simulink model "PercobaanElinKu"  (R2021a)
settings: Solver=VariableStepAuto  StartTime=0.0  StopTime=10.0  RelTol=1e-3
values from neighbouring files (symbols this model uses):
  F = 500    [JeremyElin.m]    (also in TugasElink.m = 1; UTS.m = 20; tgs.m = 20)
  k = 2000000    [JeremyElin.m]    (also in JeremyElin_K.m = 1; PercobaanElin.m = 1.3862; Riswari.m; TugasElink.m = 1)
undefined symbols (not defined in the file or in its folder): hv
libraries: pid_lib x1
settings Model: Creator=asus  LastModifiedBy=asus

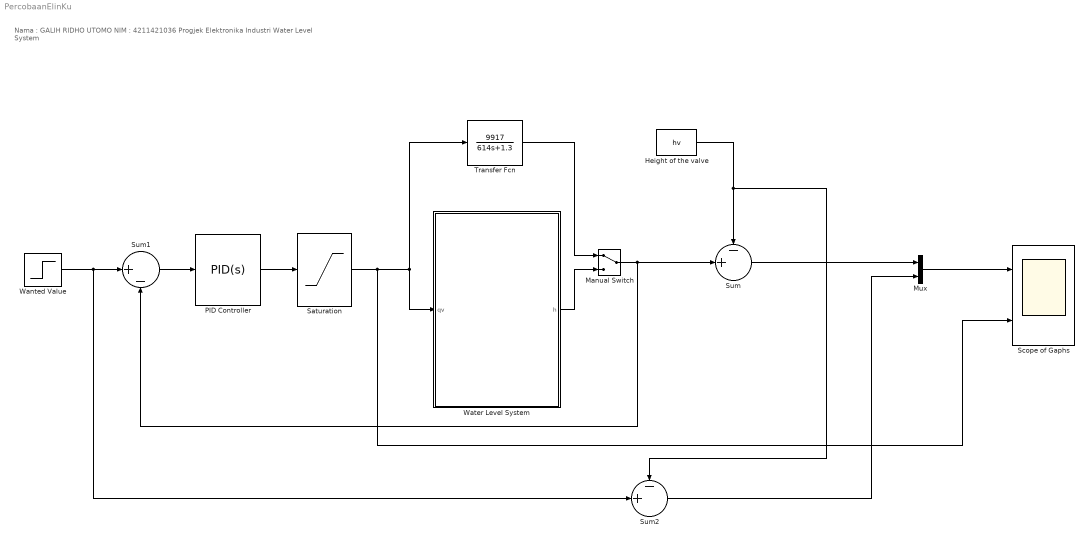
== system PercobaanElinKu ==
  note: Nama 	: GALIH RIDHO UTOMO
      | NIM 	: 4211421036
      | Progjek Elektronika Industri Water Level System
  Height of the valve : Constant  Value=hv
  Manual Switch : ManualSwitch
  Mux : Mux  Inputs=2
  PID Controller : pid_lib/PID Controller  Controller=PID  Form=Parallel  TimeDomain=Continuous-time  UseExternalTs=off  SampleTime=-1  IntegratorMethod=Forward Euler  FilterMethod=Forward Euler  ControllerParametersSource=internal  P=0.000714425130471728  I=3.53685623964158e-06  D=-0.0103917451728758  UseFilter=on  N=0.0336580030389097  TunerSelectOption=Transfer Function Based (PID Tuner App)  InitialConditionSource=internal  InitialConditionForIntegrator=0  InitialConditionForFilter=0  DifferentiatorICPrevScaledInput=0  ExternalReset=none  TrackingMode=off  Kt=1  LimitOutput=off  SatLimitsSource=internal  UpperSaturationLimit=inf  LowerSaturationLimit=-inf  LinearizeAsGain=on  AntiWindupMode=none  Kb=1  POutMin=[]  POutMax=[]  IOutMin=[]  IOutMax=[]  DOutMin=[]  DOutMax=[]  NOutMin=[]  NOutMax=[]  SumOutMin=[]  SumOutMax=[]  SaturationOutMin=[]  SaturationOutMax=[]  PParamMin=[]  PParamMax=[]  IParamMin=[]  IParamMax=[]  DParamMin=[]  DParamMax=[]  NParamMin=[]  NParamMax=[]  KbParamMin=[]  KbParamMax=[]  KtParamMin=[]  KtParamMax=[]  KbOutMin=[]  KbOutMax=[]  KtOutMin=[]  KtOutMax=[]  IntegratorOutMin=[]  IntegratorOutMax=[]  FilterOutMin=[]  FilterOutMax=[]  SumI1OutMin=[]  SumI1OutMax=[]  SumI2OutMin=[]  SumI2OutMax=[]  SumI3OutMin=[]  SumI3OutMax=[]  SumI4OutMin=[]  SumI4OutMax=[]  SumDOutMin=[]  SumDOutMax=[]  DifferentiatorOutMin=[]  DifferentiatorOutMax=[]  FilterDiffOutCoefMin=[]  FilterDiffOutCoefMax=[]  ReciprocalOutMin=[]  ReciprocalOutMax=[]  SumDenOutMin=[]  SumDenOutMax=[]  SumNumOutMin=[]  SumNumOutMax=[]  DivideOutMin=[]  DivideOutMax=[]  UdiffTsProdOutMin=[]  UdiffTsProdOutMax=[]  NTsProdOutMin=[]  NTsProdOutMax=[]  UintegralTsProdOutMin=[]  UintegralTsProdOutMax=[]  UngainTsProdOutMin=[]  UngainTsProdOutMax=[]  IntegratorContinuousStateAttributes=''  IntegratorStateMustResolveToSignalObject=off  IntegratorRTWStateStorageClass=Auto  FilterContinuousStateAttributes=''  FilterStateMustResolveToSignalObject=off  FilterRTWStateStorageClass=Auto  ParallelPVariant=InternalParameters  IdealPVariant=Disabled  IVariant=InternalParameters  DVariant=InternalParameters  IntegratorVariant=Continuous  SatVariant=Disabled  AWVariant=Passthrough  PCopyVariant=Disabled  TRVariant=Disabled  FdbkBlocksVariant=Forward  IdealPFdbkVariant=Disabled  SatFdbkVariant=Disabled  DerivativeFilterVariant=ContFilter  NVariant=InternalParameters  NCopyVariant=Disabled  FilterICVariant=InternalICsFilter  IntegratorICVariant=InternalICs  ExternalResetVariant=Disabled  TRSumVariant=Passthrough  SumFdbkVariant=Disabled  SumVariant=Sum_PID  TsampFilterVariant=InternalTs  TsampNgainVariant=Passthrough  TsampIntegralVariant=Passthrough  ExternalSaturationOutDataTypeStr=Inherit: Same as second input
  Saturation : Saturate
  Scope of Gaphs : Scope  NumInputPorts=2
  Sum : Sum  Inputs=-+|
  Sum1 : Sum  Inputs=|+-
  Sum2 : Sum  Inputs=-+|
  Transfer Fcn : TransferFcn  Numerator=[9917]  Denominator=[614 1.3]
  Wanted Value : Step  SampleTime=0
  Water Level System : Subsystem
      mask Display: image('C:\Users\asus\OneDrive - mail.unnes.ac.id\Pictures\Screenshots\Screenshot 2023-10-30 212104.png'); % Use "Edit Image" on toolstrip to change.
  wires:
  Wanted Value/1 -> Sum1/1, Sum2/2
  Sum1/1 -> PID Controller/1
  PID Controller/1 -> Saturation/1
  Saturation/1 -> Scope of Gaphs/2, Transfer Fcn/1, Water Level System/1(qv)
  Transfer Fcn/1 -> Manual Switch/1
  Water Level System/1(h) -> Manual Switch/2
  Manual Switch/1 -> Sum/2, Sum1/2
  Height of the valve/1 -> Sum2/1, Sum/1
  Sum2/1 -> Mux/2
  Sum/1 -> Mux/1
  Mux/1 -> Scope of Gaphs/1

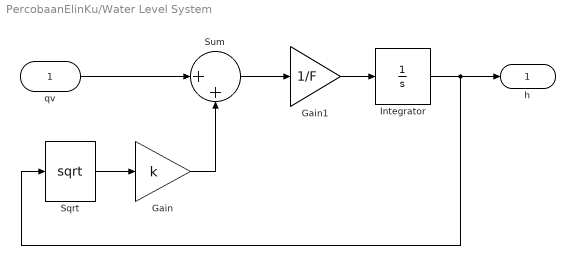
== system PercobaanElinKu/Water Level System ==
  qv : Inport
  Gain : Gain  Gain=k
  Gain1 : Gain  Gain=1/F
  Integrator : Integrator  InitialCondition=1.008*10^(-3)
  Sqrt : Sqrt  SaturateOnIntegerOverflow=on
  Sum : Sum  Inputs=|++
  h : Outport
  wires:
  Gain/1 -> Sum/2
  Sqrt/1 -> Gain/1
  Integrator/1 -> Sqrt/1, h/1
  qv/1 -> Sum/1
  Gain1/1 -> Integrator/1
  Sum/1 -> Gain1/1
